simulink model "cute_heatsys_model"  (R2018b)
settings: Solver=VariableStepAuto  StartTime=0.0  StopTime=10.0  RelTol=1e-3
undefined symbols (not defined in the file): TinHeatK, TinIC
libraries: fl_lib x21, nesl_utility x8
settings Model: Creator=Gyulai László  LastModifiedBy=Gyulai László

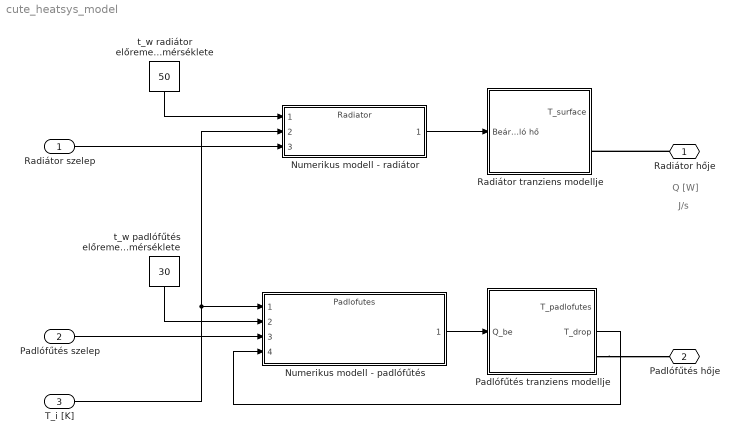
== system cute_heatsys_model ==
  note: J/s
  note: Q [W]
  Radiátor szelep : Inport
  Padlófűtés szelep : Inport  Port=2
  T_i [K] : Inport  Port=3
  Numerikus modell - padlófűtés : ModelReference  ModelNameDialog=Padlofutes.slx  SimulationMode=Normal  ModelReferenceVersion=1.28
  Numerikus modell - radiátor : ModelReference  ModelNameDialog=Radiator  SimulationMode=Normal  ModelReferenceVersion=1.30
  Padlófűtés tranziens modellje : Subsystem
  Radiátor tranziens modellje : Subsystem
  t_w padlófűtés előremenő vízhőmérséklete : Constant  Value=30
  t_w radiátor előremenő vízhőmérséklete : Constant  Value=50
  Radiátor hője : PMIOPort  Side=Right
  Padlófűtés hője : PMIOPort  Port=2  Side=Right
  wires:
  T_i [K]/1 -> Numerikus modell - radiátor/2, Numerikus modell - padlófűtés/1
  Numerikus modell - radiátor/1 -> Radiátor tranziens modellje/1(Beáramló hő)
  Padlófűtés tranziens modellje/2(T_drop) -> Numerikus modell - padlófűtés/4
  Numerikus modell - padlófűtés/1 -> Padlófűtés tranziens modellje/1(Q_be)
  Radiátor szelep/1 -> Numerikus modell - radiátor/3
  Padlófűtés szelep/1 -> Numerikus modell - padlófűtés/3
  t_w padlófűtés előremenő vízhőmérséklete/1 -> Numerikus modell - padlófűtés/2
  t_w radiátor előremenő vízhőmérséklete/1 -> Numerikus modell - radiátor/1
  connections:
  Radiátor hője/RConn1 -- Radiátor tranziens modellje/RConn1
  Padlófűtés tranziens modellje/RConn1 -- Padlófűtés hője/RConn1

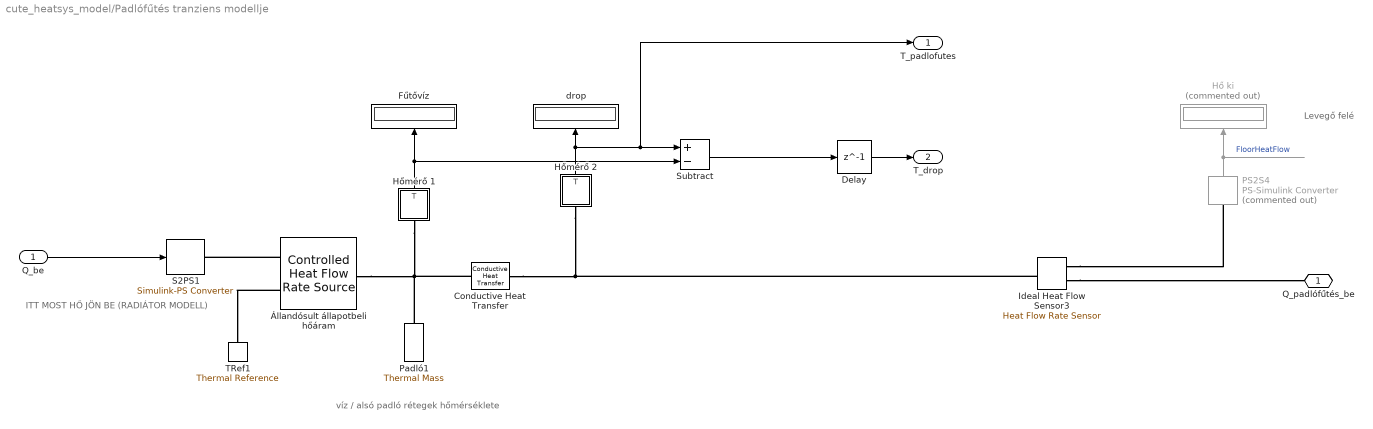
== system cute_heatsys_model/Padlófűtés tranziens modellje ==
  note: víz / alsó padló rétegek hőmérséklete
  note: ITT MOST HŐ JÖN BE (RADIÁTOR MODELL)
  note: Levegő felé
  Q_be : Inport
  Conductive Heat Transfer : fl_lib/Thermal/Thermal Elements/Conductive Heat Transfer  area=15 m^2  thickness=0.05 m  th_cond=1.2 W/(m*K)  T_specify=off  T_priority=None  T=0 K  T_nominal_specify=off  T_nominal_unit=K  T_nominal_value=1  Q_specify=off  Q_priority=None  Q=0 J/s  Q_nominal_specify=off  Q_nominal_unit=W  Q_nominal_value=1
      settings: SourceProductName=Simscape
  Delay : Delay  DelayLength=1  InitialCondition=0
  Fűtővíz : Display
  Hő ki : Display  Commented=on
  Hőmérő 1 : Subsystem
  Hőmérő 2 : Subsystem
  Ideal Heat Flow Sensor3 : fl_lib/Thermal/Thermal Sensors/Heat Flow Rate Sensor
      settings: SourceProductName=Simscape  SourceProductBaseCode=SS
  PS2S4 : nesl_utility/PS-Simulink Converter  Commented=on  PhysicalDomain=network_engine_domain  SubClassName=ps_output  LeftPortType=input  RightPortType=output  PseudoPeriodic=off  Frequencies=[]  Unit=J/s  AffineConversion=on
  Padló1 : fl_lib/Thermal/Thermal Elements/Thermal Mass  mass=1000 kg  sp_heat=840 J/kg/K  T_specify=on  T_priority=High  T=TinIC degC  T_nominal_specify=off  T_nominal_unit=K  T_nominal_value=1  Q_specify=off  Q_priority=None  Q=0 J/s  Q_nominal_specify=off  Q_nominal_unit=W  Q_nominal_value=1
      settings: LogSimulationData=on
  S2PS1 : nesl_utility/Simulink-PS Converter  PhysicalDomain=network_engine_domain  SubClassName=ps_input  LeftPortType=input  RightPortType=output  PseudoPeriodic=off  Frequencies=[]  NoiseDistribution=none  NoiseParameters=[]  Unit=1  AffineConversion=off  FilteringAndDerivatives=zero  SimscapeFilterOrder=1  InputFilterTimeConstant=.001  UdotUserProvided=0
  Subtract : Sum  Inputs=+-
  TRef1 : fl_lib/Thermal/Thermal Elements/Thermal Reference
  drop : Display
  Állandósult állapotbeli hőáram : fl_lib/Thermal/Thermal Sources/Controlled Heat Flow Rate Source
      settings: SourceProductName=Simscape
  Q_padlófűtés_be : PMIOPort  Side=Right
  T_padlofutes : Outport
  T_drop : Outport  Port=2
  wires:
  Hőmérő 1/1(T) -> Fűtővíz/1, Subtract/2
  Hőmérő 2/1(T) -> drop/1, T_padlofutes/1, Subtract/1
  Q_be/1 -> S2PS1/1
  Subtract/1 -> Delay/1
  Delay/1 -> T_drop/1
  PS2S4/1 -> Hő ki/1  "FloorHeatFlow"
  connections:
  Conductive Heat Transfer/RConn1 -- Hőmérő 2/LConn1 -- Ideal Heat Flow Sensor3/LConn1
  Conductive Heat Transfer/LConn1 -- Állandósult állapotbeli hőáram/LConn1 -- Padló1/LConn1 -- Hőmérő 1/LConn1
  Állandósult állapotbeli hőáram/RConn1 -- S2PS1/RConn1
  Állandósult állapotbeli hőáram/RConn2 -- TRef1/LConn1
  Ideal Heat Flow Sensor3/RConn2 -- Q_padlófűtés_be/RConn1
  Ideal Heat Flow Sensor3/RConn1 -- PS2S4/LConn1

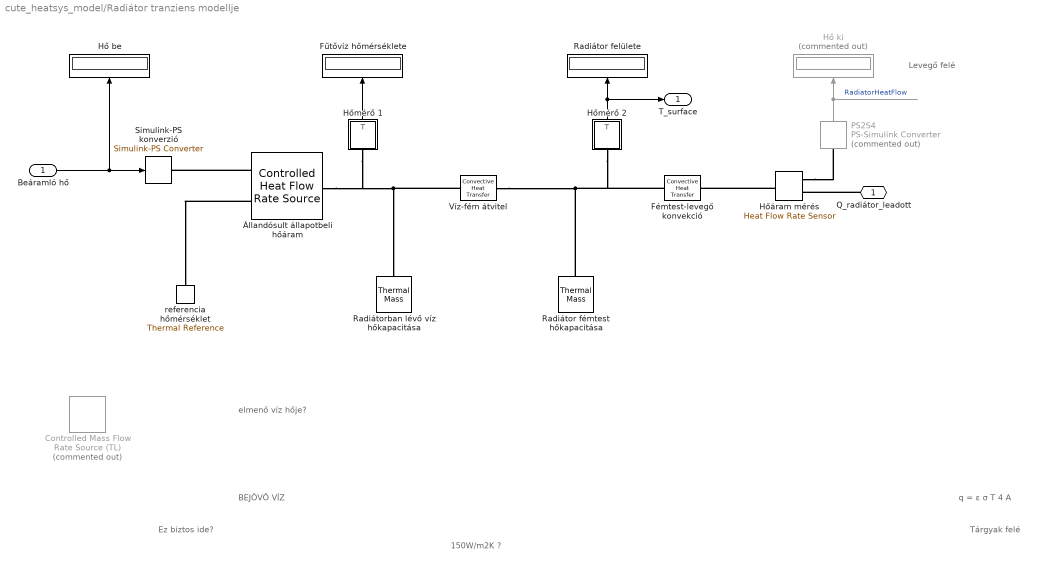
== system cute_heatsys_model/Radiátor tranziens modellje ==
  note: elmenő víz hője?
  note: BEJÖVŐ VÍZ
  note: q = ε σ T 4 A
  note: 150W/m2K ?
  note: Tárgyak felé
  note: Levegő felé
  note: Ez biztos ide?
  Beáramló hő : Inport
  Controlled Mass Flow Rate Source (TL) : fl_lib/Thermal Liquid/Sources/Controlled Mass Flow Rate Source (TL)  Commented=on  area=0.01 m^2  length=0.1 m  mdot_A_specify=off  mdot_A_priority=None  mdot_A=1 kg/s  mdot_A_nominal_specify=off  mdot_A_nominal_unit=kg/s  mdot_A_nominal_value=1
      settings: SourceProductName=Simscape  SourceProductBaseCode=SS
  Fémtest-levegő konvekció : fl_lib/Thermal/Thermal Elements/Convective Heat Transfer  area=area_radiator m^2  heat_tr_coeff=h_c_radi W/(m^2 * K)  T_specify=off  T_priority=None  T=0 K  T_nominal_specify=off  T_nominal_unit=K  T_nominal_value=1  Q_specify=off  Q_priority=None  Q=0 J/s  Q_nominal_specify=off  Q_nominal_unit=W  Q_nominal_value=1
  Fűtővíz hőmérséklete : Display
  Hő be : Display
  Hő ki : Display  Commented=on
  Hőmérő 1 : Subsystem
  Hőmérő 2 : Subsystem
  Hőáram mérés : fl_lib/Thermal/Thermal Sensors/Heat Flow Rate Sensor
      settings: SourceProductName=Simscape  SourceProductBaseCode=SS
  PS2S4 : nesl_utility/PS-Simulink Converter  Commented=on  PhysicalDomain=network_engine_domain  SubClassName=ps_output  LeftPortType=input  RightPortType=output  PseudoPeriodic=off  Frequencies=[]  Unit=J/s  AffineConversion=on
  Radiátor felülete : Display
  Radiátor fémtest hőkapacitása : fl_lib/Thermal/Thermal Elements/Thermal Mass  mass=m_r kg  sp_heat=c_metal J/kg/K  T_specify=on  T_priority=High  T=TinHeatK K  T_nominal_specify=off  T_nominal_unit=K  T_nominal_value=1  Q_specify=off  Q_priority=None  Q=0 J/s  Q_nominal_specify=off  Q_nominal_unit=W  Q_nominal_value=1
  Radiátorban lévő víz hőkapacitása : fl_lib/Thermal/Thermal Elements/Thermal Mass  mass=m_w_r kg  sp_heat=c_w J/kg/K  T_specify=on  T_priority=High  T=TinHeatK K  T_nominal_specify=off  T_nominal_unit=K  T_nominal_value=1  Q_specify=off  Q_priority=None  Q=0 J/s  Q_nominal_specify=off  Q_nominal_unit=W  Q_nominal_value=1
  Simulink-PS konverzió : nesl_utility/Simulink-PS Converter  PhysicalDomain=network_engine_domain  SubClassName=ps_input  LeftPortType=input  RightPortType=output  PseudoPeriodic=off  Frequencies=[]  NoiseDistribution=none  NoiseParameters=[]  Unit=1  AffineConversion=off  FilteringAndDerivatives=zero  SimscapeFilterOrder=1  InputFilterTimeConstant=0.001  UdotUserProvided=1
  Víz-fém átvitel : fl_lib/Thermal/Thermal Elements/Convective Heat Transfer  area=area_radiator m^2  heat_tr_coeff=h_w_radi W/(m^2 * K)  T_specify=off  T_priority=None  T=0 K  T_nominal_specify=off  T_nominal_unit=K  T_nominal_value=1  Q_specify=off  Q_priority=None  Q=0 J/s  Q_nominal_specify=off  Q_nominal_unit=W  Q_nominal_value=1
  referencia hőmérséklet : fl_lib/Thermal/Thermal Elements/Thermal Reference
  Állandósult állapotbeli hőáram : fl_lib/Thermal/Thermal Sources/Controlled Heat Flow Rate Source
      settings: SourceProductName=Simscape
  Q_radiátor_leadott : PMIOPort  Side=Right
  T_surface : Outport
  wires:
  Beáramló hő/1 -> Simulink-PS konverzió/1, Hő be/1
  Hőmérő 2/1(T) -> Radiátor felülete/1, T_surface/1
  Hőmérő 1/1(T) -> Fűtővíz hőmérséklete/1
  PS2S4/1 -> Hő ki/1  "RadiatorHeatFlow"
  connections:
  Állandósult állapotbeli hőáram/RConn1 -- Simulink-PS konverzió/RConn1
  Radiátor fémtest hőkapacitása/LConn1 -- Fémtest-levegő konvekció/LConn1 -- Hőmérő 2/LConn1 -- Víz-fém átvitel/RConn1
  Víz-fém átvitel/LConn1 -- Állandósult állapotbeli hőáram/LConn1 -- Hőmérő 1/LConn1 -- Radiátorban lévő víz hőkapacitása/LConn1
  Állandósult állapotbeli hőáram/RConn2 -- referencia hőmérséklet/LConn1
  Hőáram mérés/RConn1 -- PS2S4/LConn1
  Q_radiátor_leadott/RConn1 -- Hőáram mérés/RConn2
  Hőáram mérés/LConn1 -- Fémtest-levegő konvekció/RConn1

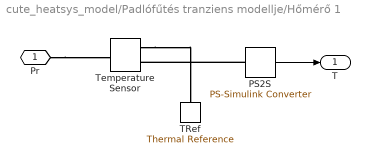
== system cute_heatsys_model/Padlófűtés tranziens modellje/Hőmérő 1 ==
  PS2S : nesl_utility/PS-Simulink Converter  PhysicalDomain=network_engine_domain  SubClassName=ps_output  LeftPortType=input  RightPortType=output  PseudoPeriodic=off  Frequencies=[]  Unit=degC  AffineConversion=on
  TRef : fl_lib/Thermal/Thermal Elements/Thermal Reference
  Temperature Sensor : fl_lib/Thermal/Thermal Sensors/Temperature Sensor
  Pr : PMIOPort  Side=Left
  T : Outport
  wires:
  PS2S/1 -> T/1
  connections:
  Temperature Sensor/RConn1 -- TRef/LConn1
  PS2S/LConn1 -- Temperature Sensor/RConn2
  Pr/RConn1 -- Temperature Sensor/LConn1

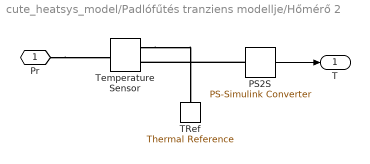
== system cute_heatsys_model/Padlófűtés tranziens modellje/Hőmérő 2 ==
  PS2S : nesl_utility/PS-Simulink Converter  PhysicalDomain=network_engine_domain  SubClassName=ps_output  LeftPortType=input  RightPortType=output  PseudoPeriodic=off  Frequencies=[]  Unit=degC  AffineConversion=on
  TRef : fl_lib/Thermal/Thermal Elements/Thermal Reference
  Temperature Sensor : fl_lib/Thermal/Thermal Sensors/Temperature Sensor
  Pr : PMIOPort  Side=Left
  T : Outport
  wires:
  PS2S/1 -> T/1
  connections:
  Temperature Sensor/RConn1 -- TRef/LConn1
  PS2S/LConn1 -- Temperature Sensor/RConn2
  Pr/RConn1 -- Temperature Sensor/LConn1

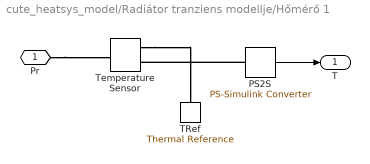
== system cute_heatsys_model/Radiátor tranziens modellje/Hőmérő 1 ==
  PS2S : nesl_utility/PS-Simulink Converter  PhysicalDomain=network_engine_domain  SubClassName=ps_output  LeftPortType=input  RightPortType=output  PseudoPeriodic=off  Frequencies=[]  Unit=degC  AffineConversion=on
  TRef : fl_lib/Thermal/Thermal Elements/Thermal Reference
  Temperature Sensor : fl_lib/Thermal/Thermal Sensors/Temperature Sensor
  Pr : PMIOPort  Side=Left
  T : Outport
  wires:
  PS2S/1 -> T/1
  connections:
  Temperature Sensor/RConn1 -- TRef/LConn1
  PS2S/LConn1 -- Temperature Sensor/RConn2
  Pr/RConn1 -- Temperature Sensor/LConn1

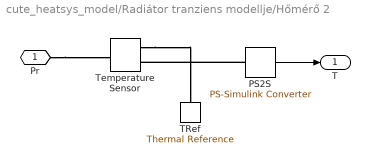
== system cute_heatsys_model/Radiátor tranziens modellje/Hőmérő 2 ==
  PS2S : nesl_utility/PS-Simulink Converter  PhysicalDomain=network_engine_domain  SubClassName=ps_output  LeftPortType=input  RightPortType=output  PseudoPeriodic=off  Frequencies=[]  Unit=degC  AffineConversion=on
  TRef : fl_lib/Thermal/Thermal Elements/Thermal Reference
  Temperature Sensor : fl_lib/Thermal/Thermal Sensors/Temperature Sensor
  Pr : PMIOPort  Side=Left
  T : Outport
  wires:
  PS2S/1 -> T/1
  connections:
  Temperature Sensor/RConn1 -- TRef/LConn1
  PS2S/LConn1 -- Temperature Sensor/RConn2
  Pr/RConn1 -- Temperature Sensor/LConn1
